simulink model "checkSetAndGetPWMs"  (R2014a)
settings: Solver=ode45  StartTime=0.0  StopTime=inf  RelTol=1e-3
libraries: WBCLibrary x3
settings Model: Creator=iron  LastModifiedBy=daniele
settings DataIOCC: SignalLoggingSaveFormat=ModelDataLogs
settings OptimizationCC: ExpressionDepthLimit=2147483647
settings DebuggingCC: UnderspecifiedInitializationDetection=Classic  FcnCallInpInsideContextMsg=UseLocalSettings  StateNameClashWarn=warning
settings GRTTargetCC: CombineOutputUpdateFcns=off  GRTInterface=on

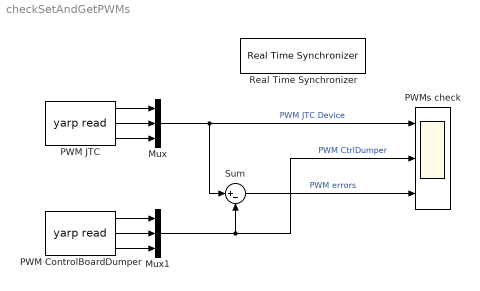
== system checkSetAndGetPWMs ==
  Mux : Mux  Inputs=3
  Mux1 : Mux  Inputs=3
  PWM ControlBoardDumper : WBCLibrary/Utilities/yarp read  from=['/controlBoardDumper/left_arm/getOutputs']  to='...'  num=3  blocking=off  timestamp=off
  PWM JTC : WBCLibrary/Utilities/yarp read  from=['/icub/jtc/left_arm/output_pwms']  to='...'  num=3  blocking=off  timestamp=off
  PWMs check : Scope  NumInputPorts=3
      settings: TimeRange=1000  YMin=-20~-20~-5  YMax=65~15~5
  Real Time Synchronizer : WBCLibrary/Utilities/Real Time Synchronizer  Priority=-10  threadPeriod=0.01
  Sum : Sum  Inputs=|+-
  wires:
  PWM JTC/2 -> Mux/2
  PWM JTC/3 -> Mux/3
  PWM JTC/1 -> Mux/1
  Mux/1 -> Sum/1, PWMs check/1  "PWM JTC Device"
  PWM ControlBoardDumper/2 -> Mux1/2
  PWM ControlBoardDumper/3 -> Mux1/3
  PWM ControlBoardDumper/1 -> Mux1/1
  Mux1/1 -> PWMs check/2, Sum/2  "PWM CtrlDumper"
  Sum/1 -> PWMs check/3  "PWM errors"
